simulink model "FarmacoCinetica"  (R2024b)
settings: Solver=ode45  StartTime=0.0  StopTime=8  FixedStep=0.01  MaxStep=1e-3  RelTol=1e-5
model workspace (MATLAB code in the model file):
  | c_gut = linspace(200,1000,5)*0.89;
  | c_1 = 0;
  | c_2= 0;
  | c_e = 0;
  | Ec_50 = 9.98;
  | E0 = 10;
  | Emax = 5.17;
  | K = 0.28;
  | k12 = 1.78;
  | k21 = 2.20;
  | Ka = 1.80;
  | ke1 = 0.83;
  | ke0 = 0.83;
  | F = 0.89;
settings Model: Creator=Miguel  LastModifiedBy=Miguel

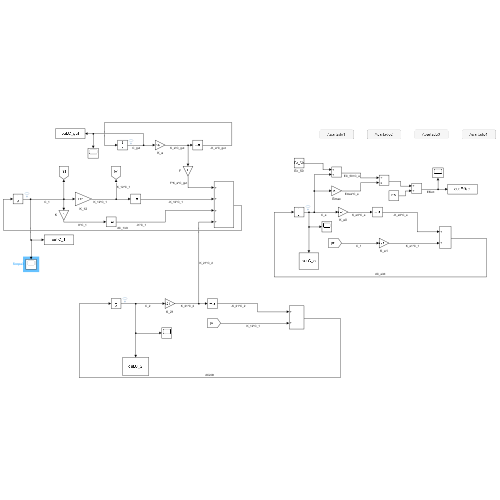
[thumbnail: Simulink's stored preview of the top-level diagram]
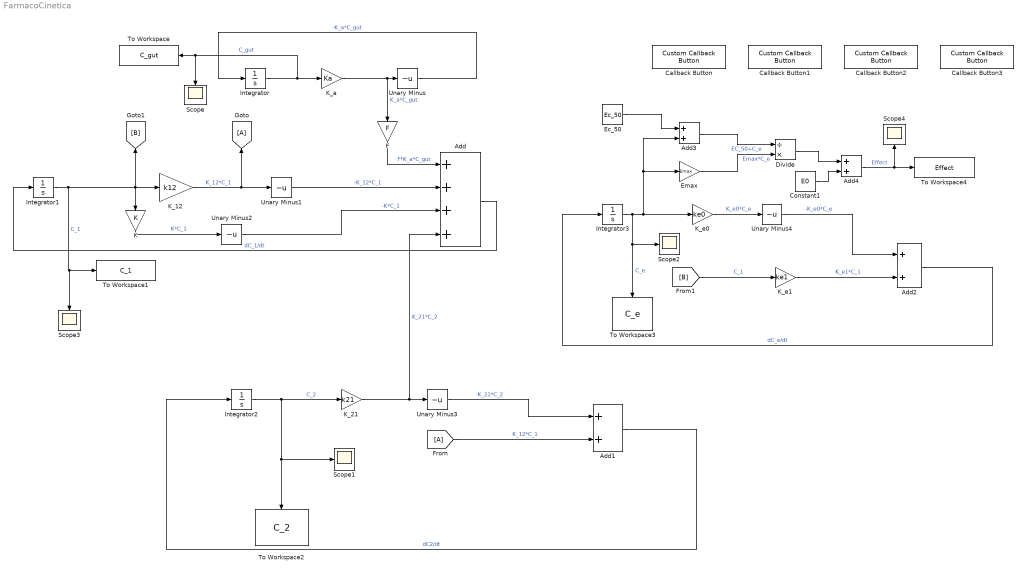
== system FarmacoCinetica ==
  Add : Sum  Inputs=++++
  Add{1..4} (4 alike) : Sum
  Callback Button : CustomCallbackButton  Configuration="{\"components\":[{\"name\":\"BackgroundImageComponent\",\"settings\":{\"image\":{\"size\":[0,0],\"src\":\"default\",\"srcOrientation\":\"Right\"},\"position\":[0,0,1,1]}},{\"name\":\"ButtonStateComponent\",\"settings\":{\"buttonType\":\"momentary\",\"clickFcn\":\"figure()\\nplot(out.tout,out.C_1,'b','LineWidth',3)\\nhold on\\nplot(out.tout,out.C_2,'r','LineWidth',3)\\nplot(out.tout,out.C_e,'g','Linewidth',3)\\nplot(out.tout,out.C_gut,'m','LineWidth',3)\\nlegend('C_1','C_2','C_e','C_{gut}')\\nxlabel('Tiempo (h)')\\nylabel('Concentración (mg\\/L)')\\ngrid on\\nhold off\\n\\nfigure()\\nplot(out.tout,out.Effect,'b','LineWidth',3)\\nxlabel('Tiempo (h)')\\nylabel('Effect')\\ngrid on\",\"onValue\":1,\"position\":[0,0,1,1],\"pressDelay\":\"500\",\"pressFcn\":\"\",\"repeatInterval\":\"0\",\"states\":[{\"horizontalAlignment\":\"center\",\"image\":{\"position\":[0,0,1,1],\"size\":[1,1],\"src\":\"default\",\"srcOrientation\":\"Right\"},\"label\":{\"color\":[0.01176470588,0.01176470588,0.01176470588,1],\"icon\":{\"size\":[0,0],\"src\":\"default\",\"srcOrientation\":\"Right\"},\"iconOffset\":0,\"iconPlacement\":\"left\",\"opacity\":1,\"show\":true,\"text\":{\"content\":\"Apartado1\",\"font\":\"Helvetica\"}},\"labelOffset\":[0,0],\"verticalAlignment\":\"middle\"},{\"horizontalAlignment\":\"center\",\"image\":{\"position\":[0,0,1,1],\"size\":[1,1],\"src\":\"default\",\"srcOrientation\":\"Right\"},\"label\":{\"color\":[0.01176470588,0.01176470588,0.01176470588,1],\"icon\":{\"size\":[0,0],\"src\":\"default\",\"srcOrientation\":\"Right\"},\"iconOffset\":0,\"iconPlacement\":\"left\",\"opacity\":1,\"show\":true,\"text\":{\"content\":\"Apartado1\",\"font\":\"Helvetica\"}},\"labelOffset\":[0,0],\"verticalAlignment\":\"middle\"},{\"horizontalAlignment\":\"center\",\"image\":{\"position\":[0,0,1,1],\"size\":[1,1],\"src\":\"default\",\"srcOrientation\":\"Right\"},\"label\":{\"color\":[0.01176470588,0.01176470588,0.01176470588,1],\"icon\":{\"size\":[0,0],\"src\":\"default\",\"srcOrientation\":\"Right\"},\"iconOffset\":0,\"iconPlacement\":\"left\",\"opacity\":1,\"show\":true,\"text\":{\"content\":\"Apartado1\",\"font\":\"Helvetica\"}},\"labelOffset\":[0,0],\"verticalAlignment\":\"middle\"},{\"horizontalAlignment\":\"center\",\"image\":{\"position\":[0,0,1,1],\"size\":[1,1],\"src\":\"default\",\"srcOrientation\":\"Right\"},\"label\":{\"color\":[0.01176470588,0.01176470588,0.01176470588,1],\"icon\":{\"size\":[0,0],\"src\":\"default\",\"srcOrientation\":\"Right\"},\"iconOffset\":0,\"iconPlacement\":\"left\",\"opacity\":1,\"show\":true,\"text\":{\"content\":\"Apartado1\",\"font\":\"Helvetica\"}},\"labelOffset\":[0,0],\"verticalAlignment\":\"middle\"}]}},{\"name\":\"ForegroundImageComponent\",\"settings\":{\"image\":{\"size\":[0,0],\"src\":\"default\",\"srcOrientation\":\"Right\"},\"isForeground\":1,\"position\":[0,0,1,1]}}],\"settings\":{\"BindingType\":\"standalone\",\"backgroundColor\":[244,244,244,1],\"backgroundOffset\":0.2,\"backgroundOpacity\":1,\"fixedAspectRatio\":\"off\",\"foregroundColor\":[0.01176470588,0.01176470588,0.01176470588,1],\"migratedFromLegacy\":true,\"useBackgroundColor\":true,\"variant\":\"callback\",\"version\":\"R2023a\"},\"type\":\"Button\"}"  CustomBackgroundColor="{\"color\":[0.9568627451,0.9568627451,0.9568627451],\"show\":true}"
  Callback Button1 : CustomCallbackButton  Configuration="{\"components\":[{\"name\":\"BackgroundImageComponent\",\"settings\":{\"image\":{\"size\":[0,0],\"src\":\"default\",\"srcOrientation\":\"Right\"},\"position\":[0,0,1,1]}},{\"name\":\"ButtonStateComponent\",\"settings\":{\"buttonType\":\"momentary\",\"clickFcn\":\"% Concentración plasmática\\nfigure()\\nplot(out.tout,out.C_1(:,1),'LineWidth',3)\\nhold on\\nfor i=2:size(out.C_1,2)\\n    plot(out.tout,out.C_1(:,i),'LineWidth',3)\\nend\\ngrid on\\nlegend('200','400','600','800','1000')\\nxlabel('Tiempo (h)')\\nylabel('Concentración plasmática (mg\\/L)')\\nhold off\\n\\n% Concentración efectiva\\nfigure()\\nplot(out.tout,out.C_e(:,1),'LineWidth',3)\\nhold on\\nfor i=2:size(out.C_e,2)\\n    plot(out.tout,out.C_e(:,i),'LineWidth',3)\\nend\\ngrid on\\nlegend('200','400','600','800','1000')\\nxlabel('Tiempo (h)')\\nylabel('Concentración efectiva (mg\\/L)')\\nhold off\",\"onValue\":1,\"position\":[0,0,1,1],\"pressDelay\":\"500\",\"pressFcn\":\"\",\"repeatInterval\":\"0\",\"states\":[{\"horizontalAlignment\":\"center\",\"image\":{\"position\":[0,0,1,1],\"size\":[1,1],\"src\":\"default\",\"srcOrientation\":\"Right\"},\"label\":{\"color\":[0.01176470588,0.01176470588,0.01176470588,1],\"icon\":{\"size\":[0,0],\"src\":\"default\",\"srcOrientation\":\"Right\"},\"iconOffset\":0,\"iconPlacement\":\"left\",\"opacity\":1,\"show\":true,\"text\":{\"content\":\"Apartado2\",\"font\":\"Helvetica\"}},\"labelOffset\":[0,0],\"verticalAlignment\":\"middle\"},{\"horizontalAlignment\":\"center\",\"image\":{\"position\":[0,0,1,1],\"size\":[1,1],\"src\":\"default\",\"srcOrientation\":\"Right\"},\"label\":{\"color\":[0.01176470588,0.01176470588,0.01176470588,1],\"icon\":{\"size\":[0,0],\"src\":\"default\",\"srcOrientation\":\"Right\"},\"iconOffset\":0,\"iconPlacement\":\"left\",\"opacity\":1,\"show\":true,\"text\":{\"content\":\"Apartado2\",\"font\":\"Helvetica\"}},\"labelOffset\":[0,0],\"verticalAlignment\":\"middle\"},{\"horizontalAlignment\":\"center\",\"image\":{\"position\":[0,0,1,1],\"size\":[1,1],\"src\":\"default\",\"srcOrientation\":\"Right\"},\"label\":{\"color\":[0.01176470588,0.01176470588,0.01176470588,1],\"icon\":{\"size\":[0,0],\"src\":\"default\",\"srcOrientation\":\"Right\"},\"iconOffset\":0,\"iconPlacement\":\"left\",\"opacity\":1,\"show\":true,\"text\":{\"content\":\"Apartado2\",\"font\":\"Helvetica\"}},\"labelOffset\":[0,0],\"verticalAlignment\":\"middle\"},{\"horizontalAlignment\":\"center\",\"image\":{\"position\":[0,0,1,1],\"size\":[1,1],\"src\":\"default\",\"srcOrientation\":\"Right\"},\"label\":{\"color\":[0.01176470588,0.01176470588,0.01176470588,1],\"icon\":{\"size\":[0,0],\"src\":\"default\",\"srcOrientation\":\"Right\"},\"iconOffset\":0,\"iconPlacement\":\"left\",\"opacity\":1,\"show\":true,\"text\":{\"content\":\"Apartado2\",\"font\":\"Helvetica\"}},\"labelOffset\":[0,0],\"verticalAlignment\":\"middle\"}]}},{\"name\":\"ForegroundImageComponent\",\"settings\":{\"image\":{\"size\":[0,0],\"src\":\"default\",\"srcOrientation\":\"Right\"},\"isForeground\":1,\"position\":[0,0,1,1]}}],\"settings\":{\"BindingType\":\"standalone\",\"backgroundColor\":[244,244,244,1],\"backgroundOffset\":0.2,\"backgroundOpacity\":1,\"fixedAspectRatio\":\"off\",\"foregroundColor\":[0.01176470588,0.01176470588,0.01176470588,1],\"migratedFromLegacy\":true,\"useBackgroundColor\":true,\"variant\":\"callback\",\"version\":\"R2023a\"},\"type\":\"Button\"}"  CustomBackgroundColor="{\"color\":[0.9568627451,0.9568627451,0.9568627451],\"show\":true}"
  Callback Button2 : CustomCallbackButton  Configuration="{\"components\":[{\"name\":\"BackgroundImageComponent\",\"settings\":{\"image\":{\"size\":[0,0],\"src\":\"default\",\"srcOrientation\":\"Right\"},\"position\":[0,0,1,1]}},{\"name\":\"ButtonStateComponent\",\"settings\":{\"buttonType\":\"momentary\",\"clickFcn\":\"% Paleta de colores\\ncolor = ['b','r','g','m','c'];\\n\\n% Concentración plasmática\\nfigure()\\nplot(out.tout,out.C_1(:,1),color(1),'LineWidth',2)\\nhold on\\nfor i=2:size(out.C_1,2)\\n    plot(out.tout,out.C_1(:,i),color(i),'LineWidth',2)\\nend\\ngrid on\\ntitle('Efecto de la tasa de eliminación')\\nlegend('0.18','0.28','0.38','0.48','0.58')\\nxlabel('Tiempo (h)')\\nylabel('Concentración plasmática (mg\\/L)')\\nhold off\\n\\n% Concentración efectiva\\nfigure()\\nplot(out.tout,out.C_e(:,1),color(1),'LineWidth',2)\\nhold on\\nfor i=2:size(out.C_e,2)\\n    plot(out.tout,out.C_e(:,i),color(i),'LineWidth',2)\\nend\\ngrid on\\ntitle('Efecto de la tasa de eliminación')\\nlegend('0.18','0.28','0.38','0.48','0.58')\\nxlabel('Tiempo (h)')\\nylabel('Concentración efectiva (mg\\/L)')\\nhold off\",\"onValue\":1,\"position\":[0,0,1,1],\"pressDelay\":\"500\",\"pressFcn\":\"\",\"repeatInterval\":\"0\",\"states\":[{\"horizontalAlignment\":\"center\",\"image\":{\"position\":[0,0,1,1],\"size\":[1,1],\"src\":\"default\",\"srcOrientation\":\"Right\"},\"label\":{\"color\":[0.01176470588,0.01176470588,0.01176470588,1],\"icon\":{\"size\":[0,0],\"src\":\"default\",\"srcOrientation\":\"Right\"},\"iconOffset\":0,\"iconPlacement\":\"left\",\"opacity\":1,\"show\":true,\"text\":{\"content\":\"Apartado3\",\"font\":\"Helvetica\"}},\"labelOffset\":[0,0],\"verticalAlignment\":\"middle\"},{\"horizontalAlignment\":\"center\",\"image\":{\"position\":[0,0,1,1],\"size\":[1,1],\"src\":\"default\",\"srcOrientation\":\"Right\"},\"label\":{\"color\":[0.01176470588,0.01176470588,0.01176470588,1],\"icon\":{\"size\":[0,0],\"src\":\"default\",\"srcOrientation\":\"Right\"},\"iconOffset\":0,\"iconPlacement\":\"left\",\"opacity\":1,\"show\":true,\"text\":{\"content\":\"Apartado3\",\"font\":\"Helvetica\"}},\"labelOffset\":[0,0],\"verticalAlignment\":\"middle\"},{\"horizontalAlignment\":\"center\",\"image\":{\"position\":[0,0,1,1],\"size\":[1,1],\"src\":\"default\",\"srcOrientation\":\"Right\"},\"label\":{\"color\":[0.01176470588,0.01176470588,0.01176470588,1],\"icon\":{\"size\":[0,0],\"src\":\"default\",\"srcOrientation\":\"Right\"},\"iconOffset\":0,\"iconPlacement\":\"left\",\"opacity\":1,\"show\":true,\"text\":{\"content\":\"Apartado3\",\"font\":\"Helvetica\"}},\"labelOffset\":[0,0],\"verticalAlignment\":\"middle\"},{\"horizontalAlignment\":\"center\",\"image\":{\"position\":[0,0,1,1],\"size\":[1,1],\"src\":\"default\",\"srcOrientation\":\"Right\"},\"label\":{\"color\":[0.01176470588,0.01176470588,0.01176470588,1],\"icon\":{\"size\":[0,0],\"src\":\"default\",\"srcOrientation\":\"Right\"},\"iconOffset\":0,\"iconPlacement\":\"left\",\"opacity\":1,\"show\":true,\"text\":{\"content\":\"Apartado3\",\"font\":\"Helvetica\"}},\"labelOffset\":[0,0],\"verticalAlignment\":\"middle\"}]}},{\"name\":\"ForegroundImageComponent\",\"settings\":{\"image\":{\"size\":[0,0],\"src\":\"default\",\"srcOrientation\":\"Right\"},\"isForeground\":1,\"position\":[0,0,1,1]}}],\"settings\":{\"BindingType\":\"standalone\",\"backgroundColor\":[244,244,244,1],\"backgroundOffset\":0.2,\"backgroundOpacity\":1,\"fixedAspectRatio\":\"off\",\"foregroundColor\":[0.01176470588,0.01176470588,0.01176470588,1],\"migratedFromLegacy\":true,\"useBackgroundColor\":true,\"variant\":\"callback\",\"version\":\"R2023a\"},\"type\":\"Button\"}"  CustomBackgroundColor="{\"color\":[0.9568627451,0.9568627451,0.9568627451],\"show\":true}"
  Callback Button3 : CustomCallbackButton  Configuration="{\"components\":[{\"name\":\"BackgroundImageComponent\",\"settings\":{\"image\":{\"size\":[0,0],\"src\":\"default\",\"srcOrientation\":\"Right\"},\"position\":[0,0,1,1]}},{\"name\":\"ButtonStateComponent\",\"settings\":{\"buttonType\":\"momentary\",\"clickFcn\":\"% Paleta de colores\\ncolor = ['b','r','g','m','c'];\\n\\n% Concentración plasmática\\nfigure()\\nplot(out.tout,out.C_1(:,1),color(1),'LineWidth',2)\\nhold on\\nfor i=2:size(out.C_1,2)\\n    plot(out.tout,out.C_1(:,i),color(i),'LineWidth',2)\\nend\\ngrid on\\ntitle('Efecto de la tasa de administración')\\nlegend('1','1.4','1.8','2.2','2.6')\\nxlabel('Tiempo (h)')\\nylabel('Concentración plasmática (mg\\/L)')\\nhold off\\n\\n% Concentración efectiva\\nfigure()\\nplot(out.tout,out.C_e(:,1),color(1),'LineWidth',2)\\nhold on\\nfor i=2:size(out.C_e,2)\\n    plot(out.tout,out.C_e(:,i),color(i),'LineWidth',2)\\nend\\ngrid on\\ntitle('Efecto de la tasa de administración')\\nlegend('1','1.4','1.8','2.2','2.6')\\nxlabel('Tiempo (h)')\\nylabel('Concentración efectiva (mg\\/L)')\\nhold off\",\"onValue\":1,\"position\":[0,0,1,1],\"pressDelay\":\"500\",\"pressFcn\":\"\",\"repeatInterval\":\"0\",\"states\":[{\"horizontalAlignment\":\"center\",\"image\":{\"position\":[0,0,1,1],\"size\":[1,1],\"src\":\"default\",\"srcOrientation\":\"Right\"},\"label\":{\"color\":[0.01176470588,0.01176470588,0.01176470588,1],\"icon\":{\"size\":[0,0],\"src\":\"default\",\"srcOrientation\":\"Right\"},\"iconOffset\":0,\"iconPlacement\":\"left\",\"opacity\":1,\"show\":true,\"text\":{\"content\":\"Apartado4\",\"font\":\"Helvetica\"}},\"labelOffset\":[0,0],\"verticalAlignment\":\"middle\"},{\"horizontalAlignment\":\"center\",\"image\":{\"position\":[0,0,1,1],\"size\":[1,1],\"src\":\"default\",\"srcOrientation\":\"Right\"},\"label\":{\"color\":[0.01176470588,0.01176470588,0.01176470588,1],\"icon\":{\"size\":[0,0],\"src\":\"default\",\"srcOrientation\":\"Right\"},\"iconOffset\":0,\"iconPlacement\":\"left\",\"opacity\":1,\"show\":true,\"text\":{\"content\":\"Apartado4\",\"font\":\"Helvetica\"}},\"labelOffset\":[0,0],\"verticalAlignment\":\"middle\"},{\"horizontalAlignment\":\"center\",\"image\":{\"position\":[0,0,1,1],\"size\":[1,1],\"src\":\"default\",\"srcOrientation\":\"Right\"},\"label\":{\"color\":[0.01176470588,0.01176470588,0.01176470588,1],\"icon\":{\"size\":[0,0],\"src\":\"default\",\"srcOrientation\":\"Right\"},\"iconOffset\":0,\"iconPlacement\":\"left\",\"opacity\":1,\"show\":true,\"text\":{\"content\":\"Apartado4\",\"font\":\"Helvetica\"}},\"labelOffset\":[0,0],\"verticalAlignment\":\"middle\"},{\"horizontalAlignment\":\"center\",\"image\":{\"position\":[0,0,1,1],\"size\":[1,1],\"src\":\"default\",\"srcOrientation\":\"Right\"},\"label\":{\"color\":[0.01176470588,0.01176470588,0.01176470588,1],\"icon\":{\"size\":[0,0],\"src\":\"default\",\"srcOrientation\":\"Right\"},\"iconOffset\":0,\"iconPlacement\":\"left\",\"opacity\":1,\"show\":true,\"text\":{\"content\":\"Apartado4\",\"font\":\"Helvetica\"}},\"labelOffset\":[0,0],\"verticalAlignment\":\"middle\"}]}},{\"name\":\"ForegroundImageComponent\",\"settings\":{\"image\":{\"size\":[0,0],\"src\":\"default\",\"srcOrientation\":\"Right\"},\"isForeground\":1,\"position\":[0,0,1,1]}}],\"settings\":{\"BindingType\":\"standalone\",\"backgroundColor\":[244,244,244,1],\"backgroundOffset\":0.2,\"backgroundOpacity\":1,\"fixedAspectRatio\":\"off\",\"foregroundColor\":[0.01176470588,0.01176470588,0.01176470588,1],\"migratedFromLegacy\":true,\"useBackgroundColor\":true,\"variant\":\"callback\",\"version\":\"R2023a\"},\"type\":\"Button\"}"  CustomBackgroundColor="{\"color\":[0.9568627451,0.9568627451,0.9568627451],\"show\":true}"
  Constant1 : Constant  Value=E0
  Divide : Product  Inputs=/*
  Ec_50 : Constant  Value=Ec_50
  Emax : Gain  Gain=Emax
  F : Gain  Gain=F
  From : From
  Goto : Goto
  Integrator : Integrator  InitialCondition=c_gut
  Integrator1 : Integrator  InitialCondition=c_1
  Integrator2 : Integrator  InitialCondition=c_2
  Integrator3 : Integrator  InitialCondition=c_e
  K : Gain  Gain=K
  K_12 : Gain  Gain=k12
  K_21 : Gain  Gain=k21
  K_a : Gain  Gain=Ka
  K_e0 : Gain  Gain=ke0
  K_e1 : Gain  Gain=ke1
  Scope{,1..4} (5 alike) : Scope
  To Workspace : ToWorkspace  VariableName=C_gut  SampleTime=-1
  To Workspace1 : ToWorkspace  VariableName=C_1  SampleTime=-1
  To Workspace2 : ToWorkspace  VariableName=C_2  SampleTime=-1
  To Workspace3 : ToWorkspace  VariableName=C_e  SampleTime=-1
  To Workspace4 : ToWorkspace  VariableName=Effect  SampleTime=-1
  Unary Minus{,1..4} (5 alike) : UnaryMinus
  wires:
  Integrator/1 -> Scope/1, To Workspace/1, K_a/1  "C_gut"
  K_a/1 -> F/1, Unary Minus/1  "K_a*C_gut"
  Unary Minus/1 -> Integrator/1  "-K_a*C_gut"
  Integrator1/1 -> Scope3/1, To Workspace1/1, [B], K/1, K_12/1  "C_1"
  K_12/1 -> Unary Minus1/1, Goto/1  "K_12*C_1"
  K/1 -> Unary Minus2/1  "K*C_1"
  F/1 -> Add/1  "F*K_a*C_gut"
  Unary Minus1/1 -> Add/2  "-K_12*C_1"
  Unary Minus2/1 -> Add/3  "-K*C_1"
  Add/1 -> Integrator1/1  "dC_1/dt"
  Integrator2/1 -> To Workspace2/1, Scope1/1, K_21/1  "C_2"
  K_21/1 -> Add/4, Unary Minus3/1  "K_21*C_2"
  Unary Minus3/1 -> Add1/1  "-K_21*C_2"
  From/1 -> Add1/2  "K_12*C_1"
  Add1/1 -> Integrator2/1  "dC2/dt"
  Integrator3/1 -> Scope2/1, To Workspace3/1, K_e0/1, Add3/2, Emax/1  "C_e"
  K_e0/1 -> Unary Minus4/1  "K_e0*C_e"
  Unary Minus4/1 -> Add2/1  "-K_e0*C_e"
  [B] -> K_e1/1  "C_1"
  K_e1/1 -> Add2/2  "K_e1*C_1"
  Add2/1 -> Integrator3/1  "dC_e/dt"
  Ec_50/1 -> Add3/1
  Add3/1 -> Divide/1  "EC_50+C_e"
  Emax/1 -> Divide/2  "Emax*C_e"
  Divide/1 -> Add4/1
  Constant1/1 -> Add4/2
  Add4/1 -> Scope4/1, To Workspace4/1  "Effect"
